simulink subsystem "Propagate_States"  (R2025b)
settings: Solver=VariableStepAuto  StartTime=0.0  StopTime=10.0  RelTol=1e-3
undefined symbols (not defined in the file): alt, g0, Ixx, Ixz, Iyy, Izz, Mass, p0, Phi0, Psi0, q0, r0, Theta0, u0, v0, w0
libraries: aerolibutil x1
settings Model: Creator=cdriggs  LastModifiedBy=cdriggs

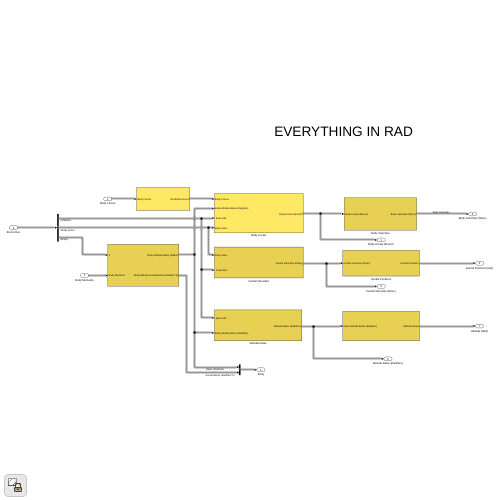
[thumbnail: Simulink's stored preview of the top-level diagram]
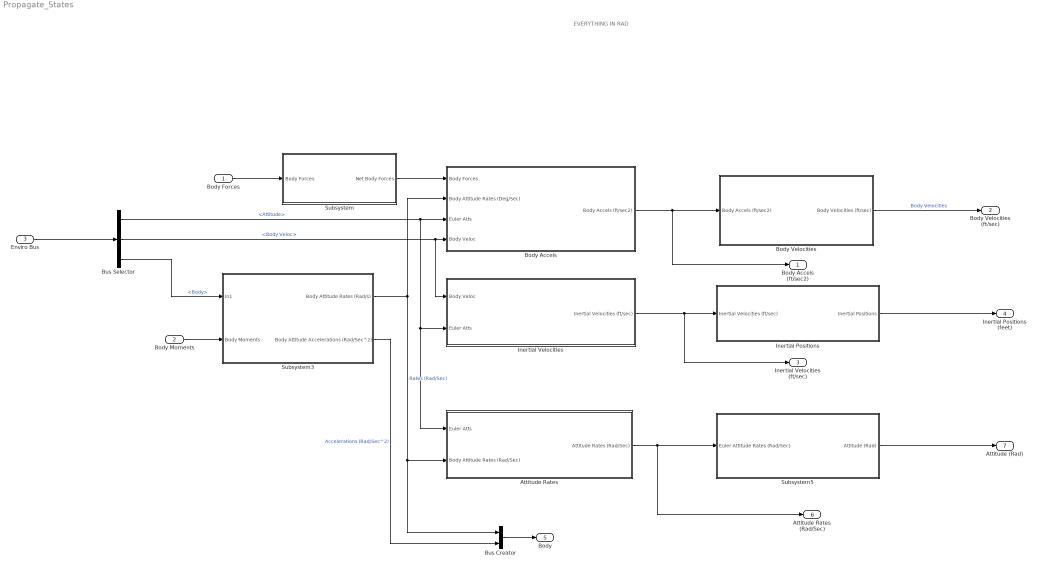
== system Propagate_States ==
  note: EVERYTHING IN RAD
  Body Forces : Inport
  Body Moments : Inport  Port=2
  Enviro Bus : Inport  Port=3
  Attitude Rates : Subsystem
  Body Accels : Subsystem
  Body Velocities : Subsystem
  Bus Creator : BusCreator  Inputs=2
  Bus Selector : BusSelector  OutputSignals=Rotat.Attitude,Trans.Body Veloc,Rotat.Body
  Inertial Positions : Subsystem
  Inertial Velocities : Subsystem
  Subsystem : Subsystem
  Subsystem3 : Subsystem
  Subsystem5 : Subsystem
  Body Accels (ft/sec2) : Outport
  Body Velocities (ft/sec) : Outport  Port=2
  Inertial Velocities (ft/sec) : Outport  Port=3
  Inertial Positions (feet) : Outport  Port=4
  " Body" : Outport  Port=5
  Attitude Rates (Rad/Sec) : Outport  Port=6
  Attitude (Rad) : Outport  Port=7
  wires:
  Bus Selector/3 -> Subsystem3/1(In1)  "<Body>"
  Bus Selector/2 -> Body Accels/4(Body Veloc), Inertial Velocities/1(Body Veloc)  "<Body Veloc>"
  Body Velocities/1(Body Velocities (ft/sec)) -> Body Velocities (ft/sec)/1  "Body Velocities"
  Subsystem3/1(Body Attitude Rates (Rad/s)) -> Body Accels/2(Body Attitude Rates (Deg/Sec)), Attitude Rates/2(Body Attitude Rates (Rad/Sec)), Bus Creator/1  "Rates (Rad/Sec)"
  Inertial Positions/1(Inertial Positions) -> Inertial Positions (feet)/1
  Inertial Velocities/1(Inertial Velocities (ft/sec)) -> Inertial Positions/1(Inertial Velocities (ft/sec)), Inertial Velocities (ft/sec)/1
  Body Accels/1(Body Accels (ft/sec2)) -> Body Velocities/1(Body Accels (ft/sec2)), Body Accels (ft/sec2)/1
  Body Moments/1 -> Subsystem3/2(Body Moments)
  Subsystem5/1(Attitude (Rad)) -> Attitude (Rad)/1
  Body Forces/1 -> Subsystem/1(Body Forces)
  Attitude Rates/1(Attitude Rates (Rad/Sec)) -> Attitude Rates (Rad/Sec)/1, Subsystem5/1(Euler Attitude Rates (Rad/Sec))
  Enviro Bus/1 -> Bus Selector/1
  Subsystem3/2(Body Attitude Accelerations (Rad/Sec^2)) -> Bus Creator/2  "Accelerations (Rad/Sec^2)"
  Subsystem/1(Net Body Forces) -> Body Accels/1(Body Forces)
  Bus Selector/1 -> Body Accels/3(" Euler Atts"), Inertial Velocities/2("  Euler Atts"), Attitude Rates/1(" Euler Atts ")  "<Attitude>"
  Bus Creator/1 -> " Body"/1

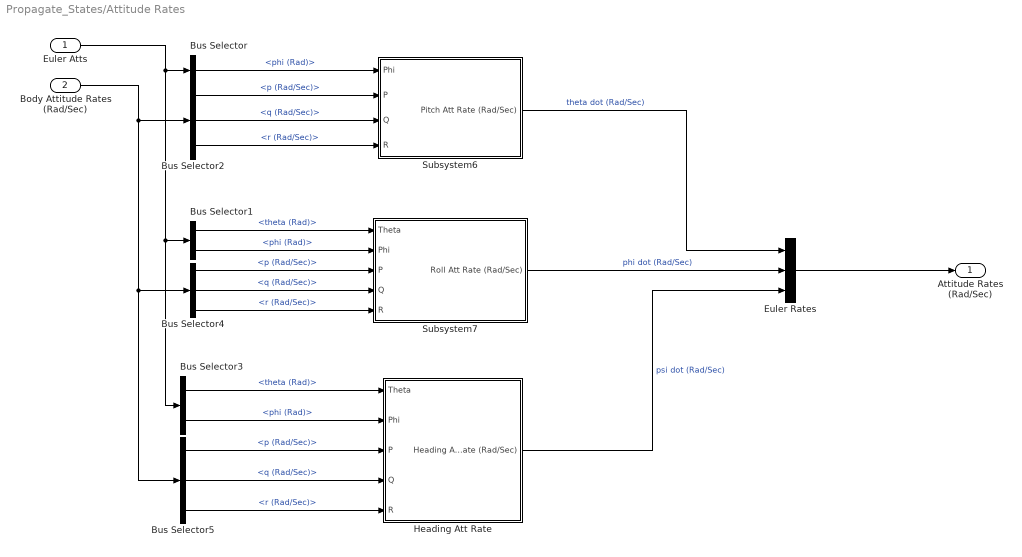
== system Propagate_States/Attitude Rates ==
  " Euler Atts " : Inport
  Body Attitude Rates (Rad/Sec) : Inport  Port=2
  Bus Selector : BusSelector  OutputSignals=phi (Rad)
  Bus Selector1 : BusSelector  OutputSignals=theta (Rad),phi (Rad)
  Bus Selector2 : BusSelector  OutputSignals=p (Rad/Sec),q (Rad/Sec),r (Rad/Sec)
  Bus Selector3 : BusSelector  OutputSignals=theta (Rad),phi (Rad)
  Bus Selector4 : BusSelector  OutputSignals=p (Rad/Sec),q (Rad/Sec),r (Rad/Sec)
  Bus Selector5 : BusSelector  OutputSignals=p (Rad/Sec),q (Rad/Sec),r (Rad/Sec)
  Euler Rates : BusCreator  Inputs=3
  Heading Att Rate : Subsystem
  Subsystem6 : Subsystem
  Subsystem7 : Subsystem
  Attitude Rates (Rad/Sec) : Outport
  wires:
  Bus Selector1/1 -> Subsystem7/1(Theta)  "<theta (Rad)>"
  Bus Selector1/2 -> Subsystem7/2(Phi)  "<phi (Rad)>"
  Bus Selector2/1 -> Subsystem6/2(P)  "<p (Rad/Sec)>"
  Bus Selector2/2 -> Subsystem6/3(Q)  "<q (Rad/Sec)>"
  Bus Selector2/3 -> Subsystem6/4(R)  "<r (Rad/Sec)>"
  Bus Selector4/1 -> Subsystem7/3(P)  "<p (Rad/Sec)>"
  Bus Selector4/2 -> Subsystem7/4(Q)  "<q (Rad/Sec)>"
  Bus Selector4/3 -> Subsystem7/5(R)  "<r (Rad/Sec)>"
  Euler Rates/1 -> Attitude Rates (Rad/Sec)/1
  Subsystem6/1(Pitch Att Rate (Rad/Sec)) -> Euler Rates/1  "theta dot (Rad/Sec)"
  Heading Att Rate/1(Heading Att Rate (Rad/Sec)) -> Euler Rates/3  "psi dot (Rad/Sec)"
  Subsystem7/1(Roll Att Rate (Rad/Sec)) -> Euler Rates/2  "phi dot (Rad/Sec)"
  Bus Selector/1 -> Subsystem6/1(Phi)  "<phi (Rad)>"
  Bus Selector3/1 -> Heading Att Rate/1(Theta)  "<theta (Rad)>"
  Bus Selector3/2 -> Heading Att Rate/2(Phi)  "<phi (Rad)>"
  " Euler Atts "/1 -> Bus Selector3/1, Bus Selector1/1, Bus Selector/1
  Bus Selector5/1 -> Heading Att Rate/3(P)  "<p (Rad/Sec)>"
  Body Attitude Rates (Rad/Sec)/1 -> Bus Selector5/1, Bus Selector4/1, Bus Selector2/1
  Bus Selector5/2 -> Heading Att Rate/4(Q)  "<q (Rad/Sec)>"
  Bus Selector5/3 -> Heading Att Rate/5(R)  "<r (Rad/Sec)>"

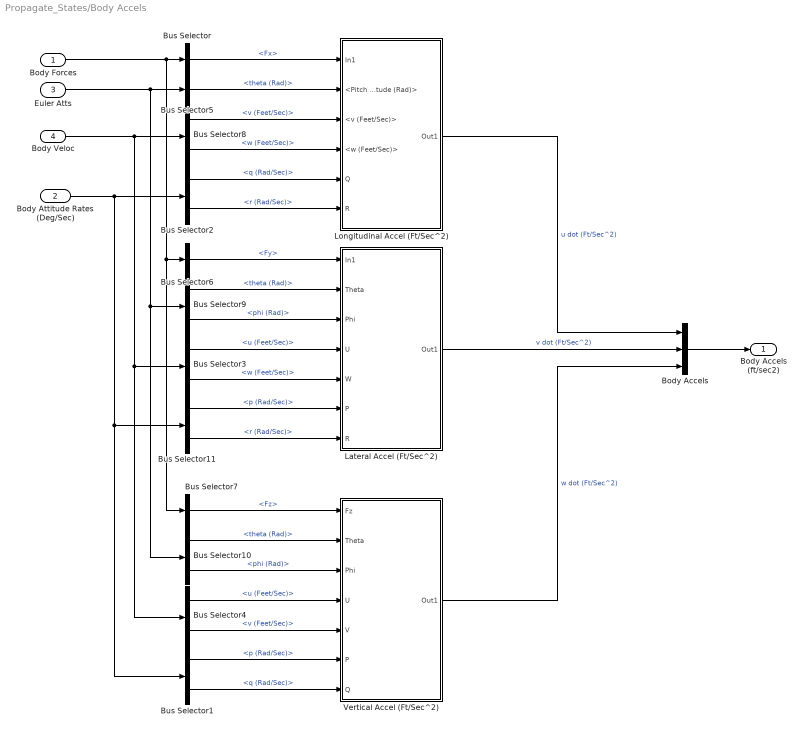
== system Propagate_States/Body Accels ==
  Body Forces : Inport
  Body Attitude Rates (Deg/Sec) : Inport  Port=2
  " Euler Atts" : Inport  Port=3
  Body Veloc : Inport  Port=4
  Body Accels : BusCreator  Inputs=3
  Bus Selector : BusSelector  OutputSignals=Fx
  Bus Selector1 : BusSelector  OutputSignals=p (Rad/Sec),q (Rad/Sec)
  Bus Selector10 : BusSelector  OutputSignals=theta (Rad),phi (Rad)
  Bus Selector11 : BusSelector  OutputSignals=p (Rad/Sec),r (Rad/Sec)
  Bus Selector2 : BusSelector  OutputSignals=q (Rad/Sec),r (Rad/Sec)
  Bus Selector3 : BusSelector  OutputSignals=u (Feet/Sec),w (Feet/Sec)
  Bus Selector4 : BusSelector  OutputSignals=u (Feet/Sec),v (Feet/Sec)
  Bus Selector5 : BusSelector  OutputSignals=theta (Rad)
  Bus Selector6 : BusSelector  OutputSignals=Fy
  Bus Selector7 : BusSelector  OutputSignals=Fz
  Bus Selector8 : BusSelector  OutputSignals=v (Feet/Sec),w (Feet/Sec)
  Bus Selector9 : BusSelector  OutputSignals=theta (Rad),phi (Rad)
  Lateral Accel (Ft/Sec^2) : Subsystem
  Longitudinal Accel (Ft/Sec^2) : Subsystem
  Vertical Accel (Ft/Sec^2) : Subsystem
  Body Accels (ft/sec2) : Outport
  wires:
  Bus Selector10/2 -> Vertical Accel (Ft/Sec^2)/3(Phi)  "<phi (Rad)>"
  Bus Selector10/1 -> Vertical Accel (Ft/Sec^2)/2(Theta)  "<theta (Rad)>"
  Bus Selector9/2 -> Lateral Accel (Ft/Sec^2)/3(Phi)  "<phi (Rad)>"
  Bus Selector9/1 -> Lateral Accel (Ft/Sec^2)/2(Theta)  "<theta (Rad)>"
  Bus Selector4/2 -> Vertical Accel (Ft/Sec^2)/5(V)  "<v (Feet/Sec)>"
  Bus Selector4/1 -> Vertical Accel (Ft/Sec^2)/4(U)  "<u (Feet/Sec)>"
  Bus Selector7/1 -> Vertical Accel (Ft/Sec^2)/1(Fz)  "<Fz>"
  Bus Selector6/1 -> Lateral Accel (Ft/Sec^2)/1(In1)  "<Fy>"
  Bus Selector3/1 -> Lateral Accel (Ft/Sec^2)/4(U)  "<u (Feet/Sec)>"
  Bus Selector3/2 -> Lateral Accel (Ft/Sec^2)/5(W)  "<w (Feet/Sec)>"
  Bus Selector8/2 -> Longitudinal Accel (Ft/Sec^2)/4(<w (Feet/Sec)>)  "<w (Feet/Sec)>"
  Bus Selector8/1 -> Longitudinal Accel (Ft/Sec^2)/3(<v (Feet/Sec)>)  "<v (Feet/Sec)>"
  Bus Selector5/1 -> Longitudinal Accel (Ft/Sec^2)/2(<Pitch Attitude (Rad)>)  "<theta (Rad)>"
  Bus Selector2/1 -> Longitudinal Accel (Ft/Sec^2)/5(Q)  "<q (Rad/Sec)>"
  Bus Selector2/2 -> Longitudinal Accel (Ft/Sec^2)/6(R)  "<r (Rad/Sec)>"
  Bus Selector1/2 -> Vertical Accel (Ft/Sec^2)/7(Q)  "<q (Rad/Sec)>"
  Bus Selector1/1 -> Vertical Accel (Ft/Sec^2)/6(P)  "<p (Rad/Sec)>"
  Body Attitude Rates (Deg/Sec)/1 -> Bus Selector11/1, Bus Selector1/1, Bus Selector2/1
  Bus Selector11/2 -> Lateral Accel (Ft/Sec^2)/7(R)  "<r (Rad/Sec)>"
  Bus Selector11/1 -> Lateral Accel (Ft/Sec^2)/6(P)  "<p (Rad/Sec)>"
  Bus Selector/1 -> Longitudinal Accel (Ft/Sec^2)/1(In1)  "<Fx>"
  Body Forces/1 -> Bus Selector/1, Bus Selector6/1, Bus Selector7/1
  " Euler Atts"/1 -> Bus Selector5/1, Bus Selector9/1, Bus Selector10/1
  Body Veloc/1 -> Bus Selector8/1, Bus Selector3/1, Bus Selector4/1
  Body Accels/1 -> Body Accels (ft/sec2)/1
  Longitudinal Accel (Ft/Sec^2)/1(Out1) -> Body Accels/1  "u dot (Ft/Sec^2)"
  Lateral Accel (Ft/Sec^2)/1(Out1) -> Body Accels/2  "v dot (Ft/Sec^2)"
  Vertical Accel (Ft/Sec^2)/1(Out1) -> Body Accels/3  "w dot (Ft/Sec^2)"

== system Propagate_States/Body Velocities ==
  Body Accels (ft/sec2) : Inport
  Body Velocities : BusCreator  Inputs=3
  Bus Selector : BusSelector  OutputSignals=u dot (Ft/Sec^2),v dot (Ft/Sec^2),w dot (Ft/Sec^2)
  Constant3 : Constant  Value=u0
  Constant4 : Constant  Value=v0
  Constant5 : Constant  Value=w0
  Integrator1 : Integrator  InitialConditionSource=external
  Integrator2 : Integrator  InitialConditionSource=external
  Integrator3 : Integrator  InitialConditionSource=external
  Pulse Generator : DiscretePulseGenerator  PulseType=Time based  Amplitude=50  Period=60  PulseWidth=5  PhaseDelay=2
  Sum : Sum  Inputs=|++
  Body Velocities (ft/sec) : Outport
  wires:
  Integrator3/1 -> Body Velocities/3  "w (Feet/Sec)"
  Pulse Generator/1 -> Sum/2
  Bus Selector/1 -> Integrator2/1  "<u dot (Ft/Sec^2)>"
  Body Accels (ft/sec2)/1 -> Bus Selector/1
  Bus Selector/2 -> Integrator1/1  "<v dot (Ft/Sec^2)>"
  Constant5/1 -> Integrator3/2
  Integrator2/1 -> Body Velocities/1  "u (Feet/Sec)"
  Constant3/1 -> Integrator2/2
  Bus Selector/3 -> Integrator3/1  "<w dot (Ft/Sec^2)>"
  Constant4/1 -> Integrator1/2
  Integrator1/1 -> Body Velocities/2  "v (Feet/Sec)"
  Body Velocities/1 -> Body Velocities (ft/sec)/1

== system Propagate_States/Inertial Positions ==
  Inertial Velocities (ft/sec) : Inport
  Bus Selector : BusSelector  OutputSignals=North-South Velocity (Feet/Sec),East-West Velocity (Feet/Sec),Inertial Vertical Speed (Feet/Sec)
  Constant : Constant  Value=0
  Constant1 : Constant  Value=0
  Constant2 : Constant  Value=-alt
  Inertial Positions ft : BusCreator  Inputs=3
  Integrator6 : Integrator  InitialConditionSource=external
  Integrator8 : Integrator  InitialConditionSource=external
  Integrator9 : Integrator  InitialConditionSource=external
  Inertial Positions : Outport
  wires:
  Constant1/1 -> Integrator8/2
  Constant/1 -> Integrator6/2
  Integrator8/1 -> Inertial Positions ft/2  "Longitude (Feet)"
  Inertial Positions ft/1 -> Inertial Positions/1
  Integrator6/1 -> Inertial Positions ft/1  "Latitude (Feet)"
  Inertial Velocities (ft/sec)/1 -> Bus Selector/1
  Bus Selector/1 -> Integrator6/1  "<North-South Velocity (Feet/Sec)>"
  Bus Selector/2 -> Integrator8/1  "<East-West Velocity (Feet/Sec)>"
  Bus Selector/3 -> Integrator9/1  "<Inertial Vertical Speed (Feet/Sec)>"
  Integrator9/1 -> Inertial Positions ft/3  "Inertial Altitude (Feet)"
  Constant2/1 -> Integrator9/2  "Inertial Altitude (Feet)"

== system Propagate_States/Inertial Velocities ==
  Body Veloc : Inport
  "  Euler Atts" : Inport  Port=2
  Bus Selector : BusSelector  OutputSignals=phi (Rad),theta (Rad),psi (Rad)
  Bus Selector1 : BusSelector  OutputSignals=phi (Rad),theta (Rad),psi (Rad)
  Bus Selector2 : BusSelector  OutputSignals=phi (Rad),theta (Rad)
  Bus Selector3 : BusSelector  OutputSignals=u (Feet/Sec),v (Feet/Sec),w (Feet/Sec)
  Bus Selector4 : BusSelector  OutputSignals=u (Feet/Sec),v (Feet/Sec),w (Feet/Sec)
  Bus Selector5 : BusSelector  OutputSignals=u (Feet/Sec),v (Feet/Sec),w (Feet/Sec)
  East-West Velocity (Feet/Sec) : Subsystem
  Inertial Velocities : BusCreator  Inputs=3
  Inertial Vertical Speed (Feet/Sec) : Subsystem
  North-South Velocity (Feet/Sec) : Subsystem
  Inertial Velocities (ft/sec) : Outport
  wires:
  "  Euler Atts"/1 -> Bus Selector2/1, Bus Selector1/1, Bus Selector/1
  Bus Selector/1 -> North-South Velocity (Feet/Sec)/1(Phi)  "<phi (Rad)>"
  Bus Selector/2 -> North-South Velocity (Feet/Sec)/2(Theta)  "<theta (Rad)>"
  Bus Selector/3 -> North-South Velocity (Feet/Sec)/3(Psi)  "<psi (Rad)>"
  Bus Selector1/1 -> East-West Velocity (Feet/Sec)/1(Phi)  "<phi (Rad)>"
  Bus Selector1/2 -> East-West Velocity (Feet/Sec)/2(Theta)  "<theta (Rad)>"
  Bus Selector1/3 -> East-West Velocity (Feet/Sec)/3(Psi)  "<psi (Rad)>"
  Bus Selector2/1 -> Inertial Vertical Speed (Feet/Sec)/1(Phi)  "<phi (Rad)>"
  Bus Selector2/2 -> Inertial Vertical Speed (Feet/Sec)/2(Theta)  "<theta (Rad)>"
  Body Veloc/1 -> Bus Selector5/1, Bus Selector4/1, Bus Selector3/1
  Bus Selector3/1 -> North-South Velocity (Feet/Sec)/4(U)  "<u (Feet/Sec)>"
  Bus Selector3/2 -> North-South Velocity (Feet/Sec)/5(V)  "<v (Feet/Sec)>"
  Bus Selector3/3 -> North-South Velocity (Feet/Sec)/6(W)  "<w (Feet/Sec)>"
  Bus Selector4/1 -> East-West Velocity (Feet/Sec)/4(U)  "<u (Feet/Sec)>"
  Bus Selector4/2 -> East-West Velocity (Feet/Sec)/5(V)  "<v (Feet/Sec)>"
  Bus Selector4/3 -> East-West Velocity (Feet/Sec)/6(W)  "<w (Feet/Sec)>"
  Bus Selector5/1 -> Inertial Vertical Speed (Feet/Sec)/3(U)  "<u (Feet/Sec)>"
  Bus Selector5/2 -> Inertial Vertical Speed (Feet/Sec)/4(V)  "<v (Feet/Sec)>"
  Bus Selector5/3 -> Inertial Vertical Speed (Feet/Sec)/5(W)  "<w (Feet/Sec)>"
  Inertial Velocities/1 -> Inertial Velocities (ft/sec)/1
  North-South Velocity (Feet/Sec)/1(North-South Velocity (Feet/Sec)) -> Inertial Velocities/1  "North-South Velocity (Feet/Sec)"
  East-West Velocity (Feet/Sec)/1(East-West Velocity (Feet/Sec)) -> Inertial Velocities/2  "East-West Velocity (Feet/Sec)"
  Inertial Vertical Speed (Feet/Sec)/1(Inertial Vertical Speed (Feet/Sec)) -> Inertial Velocities/3  "Inertial Vertical Speed (Feet/Sec)"

== system Propagate_States/Subsystem ==
  Body Forces : Inport
  Add1 : Sum
  Add2 : Sum
  Add3 : Sum
  Bus Creator : BusCreator  Inputs=3
  Bus Selector2 : BusSelector  OutputSignals=FAX (Lb),FTX (Lb),FAY (Lb),FTY (Lb),FAZ (Lb),FTZ (Lb)
  Net Body Forces : Outport
  wires:
  Add3/1 -> Bus Creator/3  "Fz"
  Bus Creator/1 -> Net Body Forces/1  "Net Body Forces"
  Bus Selector2/6 -> Add3/2  "<FTZ (Lb)>"
  Bus Selector2/5 -> Add3/1  "<FAZ (Lb)>"
  Bus Selector2/2 -> Add2/2  "<FTX (Lb)>"
  Bus Selector2/1 -> Add2/1  "<FAX (Lb)>"
  Add1/1 -> Bus Creator/2  "Fy"
  Add2/1 -> Bus Creator/1  "Fx"
  Bus Selector2/4 -> Add1/2  "<FTY (Lb)>"
  Body Forces/1 -> Bus Selector2/1
  Bus Selector2/3 -> Add1/1  "<FAY (Lb)>"

== system Propagate_States/Subsystem3 ==
  In1 : Inport
  Body Moments : Inport  Port=2
  Bus Selector9 : BusSelector  OutputSignals=Rates (Rad/Sec).p (Rad/Sec),Rates (Rad/Sec).q (Rad/Sec),Rates (Rad/Sec).r (Rad/Sec)
  Constant : Constant  Value=[Ixx 0 -Ixz; 0 Iyy 0; -Ixz 0 Izz]
  Invert 3x3 Matrix : aerolibutil/Invert  3x3 Matrix
  Make Vector 1 : Concatenate  NumInputs=3
  Make vector rows : Subsystem
  MatrixMultiply : Product  Multiplication=Matrix(*)
  Subsystem1 : Subsystem
  Subsystem4 : Subsystem
  Subsystem5 : Subsystem
  Body Attitude Rates (Rad/s) : Outport
  Body Attitude Accelerations (Rad/Sec^2) : Outport  Port=2
  wires:
  Body Moments/1 -> Subsystem5/1(Body Moments)
  Bus Selector9/3 -> Subsystem4/3(<Yaw Rate (Rad/Sec)>)  "<r (Rad/Sec)>"
  Bus Selector9/2 -> Subsystem4/2(<Pitch Rate (Rad/Sec)>)  "<q (Rad/Sec)>"
  Bus Selector9/1 -> Subsystem4/1(<Roll Rate (Rad/Sec)>)  "<p (Rad/Sec)>"
  Constant/1 -> Invert 3x3 Matrix/1
  In1/1 -> Bus Selector9/1
  Invert 3x3 Matrix/1 -> MatrixMultiply/1
  Make vector rows/1(Out1) -> Make Vector 1/1
  Make vector rows/2(Out2) -> Make Vector 1/2
  Make vector rows/3(Out3) -> Make Vector 1/3
  Make Vector 1/1 -> MatrixMultiply/2
  Subsystem4/3(QR) -> Make vector rows/3(QR)
  Subsystem4/4((P^2-R^2)) -> Make vector rows/4((P^2-R^2))
  Subsystem4/2(PR) -> Make vector rows/2(PR)
  Subsystem4/1(PQ) -> Make vector rows/1(PQ)
  Subsystem1/2(Body Attitude Accelerations (Rad/Sec^2)) -> Body Attitude Accelerations (Rad/Sec^2)/1
  Subsystem1/1(Body Attitude Rates (Rad/Sec)) -> Body Attitude Rates (Rad/s)/1
  MatrixMultiply/1 -> Subsystem1/1(In1)
  Subsystem5/1(Net Body Moments) -> Make vector rows/5(Net Body Moments)

== system Propagate_States/Subsystem5 ==
  Euler Attitude Rates (Rad/Sec) : Inport
  Bus Selector : BusSelector  OutputSignals=phi dot (Rad/Sec),theta dot (Rad/Sec),psi dot (Rad/Sec)
  Constant12 : Constant  Value=Psi0
  Constant14 : Constant  Value=Phi0
  Constant7 : Constant  Value=Theta0
  Euler Attitudes : BusCreator  Inputs=3
  Integrator4 : Integrator  InitialConditionSource=external
  Integrator5 : Integrator  InitialConditionSource=external
  Integrator7 : Integrator  InitialConditionSource=external
  Attitude (Rad) : Outport
  wires:
  Integrator5/1 -> Euler Attitudes/2  "theta (Rad)"
  Constant12/1 -> Integrator4/2
  Constant14/1 -> Integrator7/2
  Euler Attitude Rates (Rad/Sec)/1 -> Bus Selector/1
  Bus Selector/1 -> Integrator7/1  "<phi dot (Rad/Sec)>"
  Bus Selector/2 -> Integrator5/1  "<theta dot (Rad/Sec)>"
  Bus Selector/3 -> Integrator4/1  "<psi dot (Rad/Sec)>"
  Euler Attitudes/1 -> Attitude (Rad)/1
  Integrator4/1 -> Euler Attitudes/3  "psi (Rad)"
  Integrator7/1 -> Euler Attitudes/1  "phi (Rad)"
  Constant7/1 -> Integrator5/2

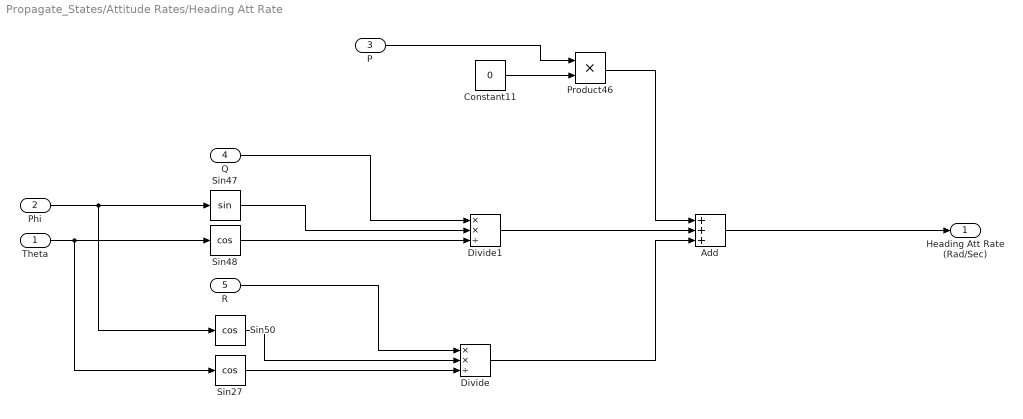
== system Propagate_States/Attitude Rates/Heading Att Rate ==
  Theta : Inport
  Phi : Inport  Port=2
  P : Inport  Port=3
  Q : Inport  Port=4
  R : Inport  Port=5
  Add : Sum  Inputs=+++
  Constant11 : Constant  Value=0
  Divide : Product  Inputs=**/
  Divide1 : Product  Inputs=**/
  Product46 : Product
  Sin27 : Trigonometry  Operator=cos
  Sin47 : Trigonometry
  Sin48 : Trigonometry  Operator=cos
  Sin50 : Trigonometry  Operator=cos
  Heading Att Rate (Rad/Sec) : Outport
  wires:
  Constant11/1 -> Product46/2
  Divide1/1 -> Add/2
  Divide/1 -> Add/3
  Sin50/1 -> Divide/2
  Sin48/1 -> Divide1/3
  Product46/1 -> Add/1
  Sin47/1 -> Divide1/2
  Sin27/1 -> Divide/3
  P/1 -> Product46/1
  Phi/1 -> Sin50/1, Sin47/1
  Theta/1 -> Sin27/1, Sin48/1
  R/1 -> Divide/1
  Add/1 -> Heading Att Rate (Rad/Sec)/1
  Q/1 -> Divide1/1

== system Propagate_States/Attitude Rates/Subsystem6 ==
  note: phi
  Phi : Inport
  P : Inport  Port=2
  Q : Inport  Port=3
  R : Inport  Port=4
  Add : Sum  Inputs=+++
  Constant9 : Constant  Value=0
  Gain : Gain  Gain=-1
  Product38 : Product
  Product39 : Product
  Product42 : Product
  Sin25 : Trigonometry  Operator=cos
  Sin26 : Trigonometry
  Pitch Att Rate (Rad/Sec) : Outport
  wires:
  Sin25/1 -> Product39/2
  Sin26/1 -> Gain/1
  Product42/1 -> Add/3
  Product38/1 -> Add/1
  Constant9/1 -> Product38/1
  Product39/1 -> Add/2
  P/1 -> Product38/2
  Q/1 -> Product39/1
  Phi/1 -> Sin26/1, Sin25/1
  R/1 -> Product42/1
  Add/1 -> Pitch Att Rate (Rad/Sec)/1  "Roll Att Rate (Rad/Sec)"
  Gain/1 -> Product42/2

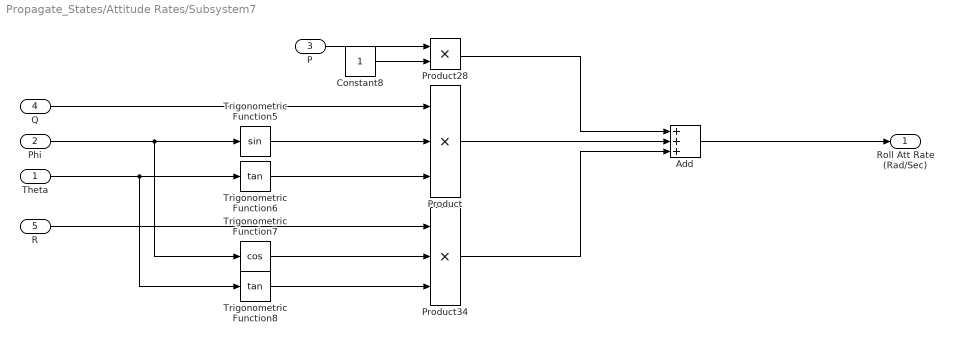
== system Propagate_States/Attitude Rates/Subsystem7 ==
  Theta : Inport
  Phi : Inport  Port=2
  P : Inport  Port=3
  Q : Inport  Port=4
  R : Inport  Port=5
  Add : Sum  Inputs=+++
  Constant8 : Constant
  Product : Product  Inputs=3
  Product28 : Product
  Product34 : Product  Inputs=3
  Trigonometric Function5 : Trigonometry
  Trigonometric Function6 : Trigonometry  Operator=tan
  Trigonometric Function7 : Trigonometry  Operator=cos
  Trigonometric Function8 : Trigonometry  Operator=tan
  Roll Att Rate (Rad/Sec) : Outport
  wires:
  Phi/1 -> Trigonometric Function7/1, Trigonometric Function5/1
  Theta/1 -> Trigonometric Function8/1, Trigonometric Function6/1
  P/1 -> Product28/1
  Product/1 -> Add/2
  Trigonometric Function8/1 -> Product34/3
  Trigonometric Function6/1 -> Product/3
  Constant8/1 -> Product28/2
  Product34/1 -> Add/3
  Trigonometric Function7/1 -> Product34/2
  R/1 -> Product34/1
  Trigonometric Function5/1 -> Product/2
  Product28/1 -> Add/1
  Add/1 -> Roll Att Rate (Rad/Sec)/1
  Q/1 -> Product/1

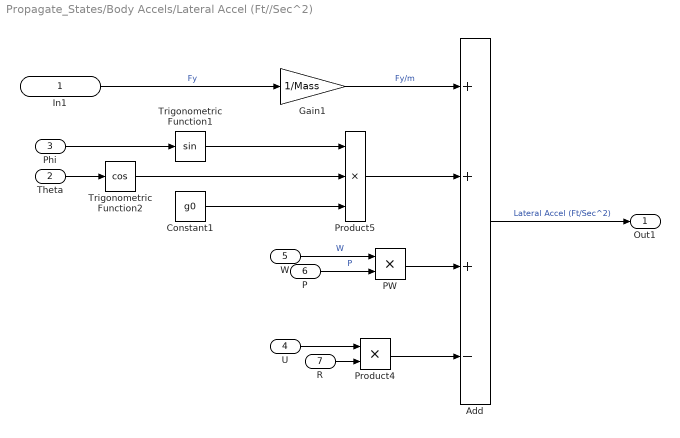
== system Propagate_States/Body Accels/Lateral Accel (Ft//Sec^2) ==
  In1 : Inport
  Theta : Inport  Port=2
  Phi : Inport  Port=3
  U : Inport  Port=4
  W : Inport  Port=5
  P : Inport  Port=6
  R : Inport  Port=7
  Add : Sum  Inputs=+++-
  Constant1 : Constant  Value=g0
  Gain1 : Gain  Gain=1/Mass
  PW : Product
  Product4 : Product
  Product5 : Product  Inputs=3
  Trigonometric Function1 : Trigonometry
  Trigonometric Function2 : Trigonometry  Operator=cos
  Out1 : Outport
  wires:
  Product5/1 -> Add/2
  Trigonometric Function1/1 -> Product5/1
  PW/1 -> Add/3
  Constant1/1 -> Product5/3
  In1/1 -> Gain1/1  "Fy"
  Trigonometric Function2/1 -> Product5/2
  Add/1 -> Out1/1  "Lateral Accel (Ft/Sec^2)"
  Product4/1 -> Add/4
  Phi/1 -> Trigonometric Function1/1
  Theta/1 -> Trigonometric Function2/1
  W/1 -> PW/1  "W"
  P/1 -> PW/2  "P"
  U/1 -> Product4/1
  R/1 -> Product4/2
  Gain1/1 -> Add/1  "Fy/m"

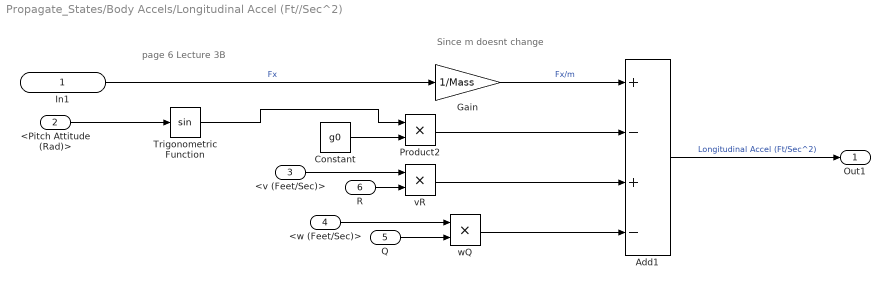
== system Propagate_States/Body Accels/Longitudinal Accel (Ft//Sec^2) ==
  note: page 6 Lecture 3B
  note: Since m doesnt change
  In1 : Inport
  <Pitch Attitude (Rad)> : Inport  Port=2
  <v (Feet/Sec)> : Inport  Port=3
  <w (Feet/Sec)> : Inport  Port=4
  Q : Inport  Port=5
  R : Inport  Port=6
  Add1 : Sum  Inputs=+-+-
  Constant : Constant  Value=g0
  Gain : Gain  Gain=1/Mass
  Product2 : Product
  Trigonometric Function : Trigonometry
  vR : Product
  wQ : Product
  Out1 : Outport
  wires:
  <Pitch Attitude (Rad)>/1 -> Trigonometric Function/1
  Trigonometric Function/1 -> Product2/1
  vR/1 -> Add1/3
  Gain/1 -> Add1/1  "Fx/m"
  Constant/1 -> Product2/2
  wQ/1 -> Add1/4
  In1/1 -> Gain/1  "Fx"
  Product2/1 -> Add1/2
  Add1/1 -> Out1/1  "Longitudinal Accel (Ft/Sec^2)"
  <v (Feet/Sec)>/1 -> vR/1
  R/1 -> vR/2
  <w (Feet/Sec)>/1 -> wQ/1
  Q/1 -> wQ/2

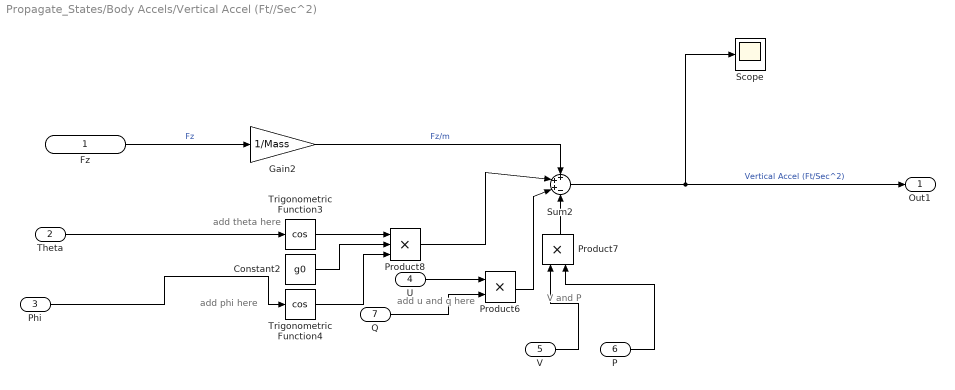
== system Propagate_States/Body Accels/Vertical Accel (Ft//Sec^2) ==
  note: add theta here
  note: V and P
  note: add u and q here
  note: add phi here
  Fz : Inport
  Theta : Inport  Port=2
  Phi : Inport  Port=3
  U : Inport  Port=4
  V : Inport  Port=5
  P : Inport  Port=6
  Q : Inport  Port=7
  Constant2 : Constant  Value=g0
  Gain2 : Gain  Gain=1/Mass
  Product6 : Product
  Product7 : Product
  Product8 : Product  Inputs=3
  Scope : Scope
      settings: ActiveDisplayYMinimum=-17.94081319561279  ActiveDisplayYMaximum=11.502802243959533  DataLoggingVariableName=ScopeData10
  Sum2 : Sum  Inputs=+++-
  Trigonometric Function3 : Trigonometry  Operator=cos
  Trigonometric Function4 : Trigonometry  Operator=cos
  Out1 : Outport
  wires:
  Fz/1 -> Gain2/1  "Fz"
  Constant2/1 -> Product8/2
  Product8/1 -> Sum2/2
  Product6/1 -> Sum2/3
  Trigonometric Function4/1 -> Product8/3
  Trigonometric Function3/1 -> Product8/1
  Gain2/1 -> Sum2/1  "Fz/m"
  Sum2/1 -> Out1/1, Scope/1  "Vertical Accel (Ft/Sec^2)"
  Product7/1 -> Sum2/4
  Theta/1 -> Trigonometric Function3/1
  Phi/1 -> Trigonometric Function4/1
  U/1 -> Product6/1
  Q/1 -> Product6/2
  V/1 -> Product7/1
  P/1 -> Product7/2

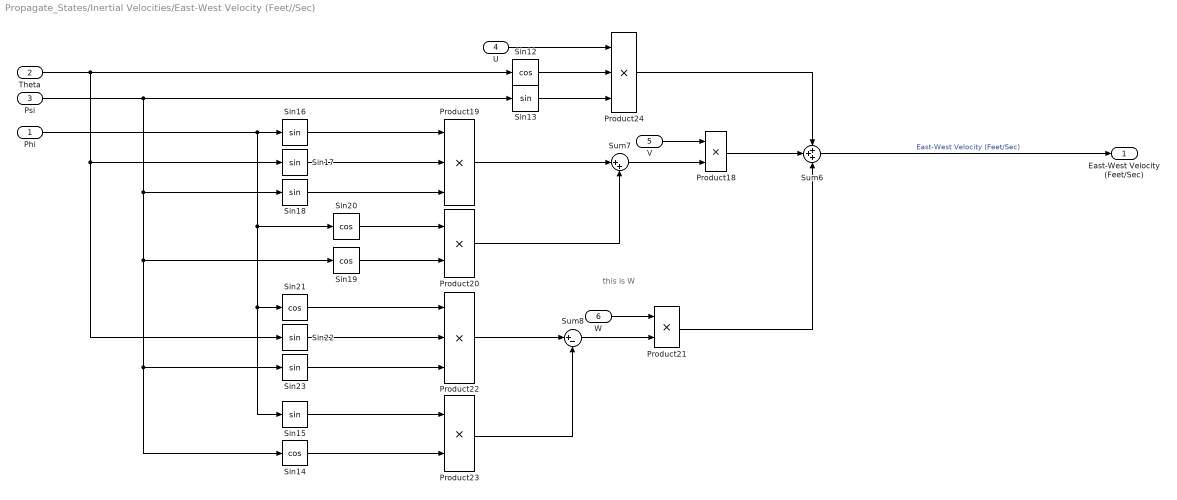
== system Propagate_States/Inertial Velocities/East-West Velocity (Feet//Sec) ==
  note: this is W
  Phi : Inport
  Theta : Inport  Port=2
  Psi : Inport  Port=3
  U : Inport  Port=4
  V : Inport  Port=5
  W : Inport  Port=6
  Product{18,20..21,23} (4 alike) : Product
  Product19 : Product  Inputs=3
  Product22 : Product  Inputs=3
  Product24 : Product  Inputs=3
  Sin{12,14,19..21} (5 alike) : Trigonometry  Operator=cos
  Sin{13,15..18,22..23} (7 alike) : Trigonometry
  Sum6 : Sum  Inputs=+++
  Sum7 : Sum  Inputs=|++
  Sum8 : Sum  Inputs=|+-
  East-West Velocity (Feet/Sec) : Outport
  wires:
  Sin14/1 -> Product23/2
  Sin17/1 -> Product19/2
  Sin15/1 -> Product23/1
  Product24/1 -> Sum6/1
  Product19/1 -> Sum7/1
  Sin22/1 -> Product22/2
  Product20/1 -> Sum7/2
  Product23/1 -> Sum8/2
  Sin16/1 -> Product19/1
  Sum7/1 -> Product18/2
  Sin12/1 -> Product24/2
  Product18/1 -> Sum6/2
  Sin23/1 -> Product22/3
  Sum8/1 -> Product21/2
  Product21/1 -> Sum6/3
  Sin21/1 -> Product22/1
  Product22/1 -> Sum8/1
  Sin13/1 -> Product24/3
  Sin18/1 -> Product19/3
  Sin19/1 -> Product20/2
  Sin20/1 -> Product20/1
  Sum6/1 -> East-West Velocity (Feet/Sec)/1  "East-West Velocity (Feet/Sec)"
  Phi/1 -> Sin21/1, Sin15/1, Sin20/1, Sin16/1
  Theta/1 -> Sin22/1, Sin17/1, Sin12/1
  Psi/1 -> Sin14/1, Sin23/1, Sin19/1, Sin18/1, Sin13/1
  U/1 -> Product24/1
  V/1 -> Product18/1
  W/1 -> Product21/1

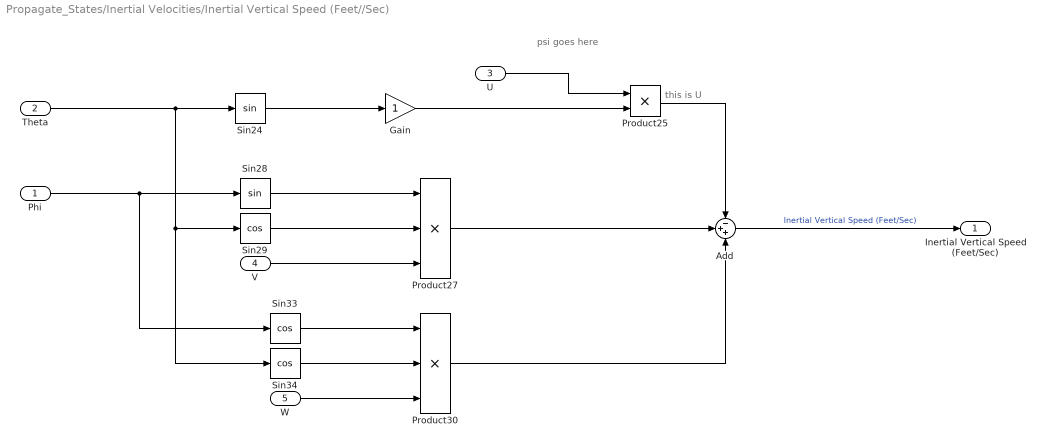
== system Propagate_States/Inertial Velocities/Inertial Vertical Speed (Feet//Sec) ==
  note: this is U
  note: psi goes here
  Phi : Inport
  Theta : Inport  Port=2
  U : Inport  Port=3
  V : Inport  Port=4
  W : Inport  Port=5
  Add : Sum  Inputs=-++
  Gain : Gain
  Product25 : Product
  Product27 : Product  Inputs=3
  Product30 : Product  Inputs=3
  Sin24 : Trigonometry
  Sin28 : Trigonometry
  Sin29 : Trigonometry  Operator=cos
  Sin33 : Trigonometry  Operator=cos
  Sin34 : Trigonometry  Operator=cos
  Inertial Vertical Speed (Feet/Sec) : Outport
  wires:
  Sin24/1 -> Gain/1
  Product30/1 -> Add/3
  Product25/1 -> Add/1
  Sin34/1 -> Product30/2
  Sin29/1 -> Product27/2
  Sin28/1 -> Product27/1
  Product27/1 -> Add/2
  Sin33/1 -> Product30/1
  Add/1 -> Inertial Vertical Speed (Feet/Sec)/1  "Inertial Vertical Speed (Feet/Sec)"
  Theta/1 -> Sin34/1, Sin29/1, Sin24/1
  Phi/1 -> Sin33/1, Sin28/1
  U/1 -> Product25/1
  W/1 -> Product30/3
  V/1 -> Product27/3
  Gain/1 -> Product25/2

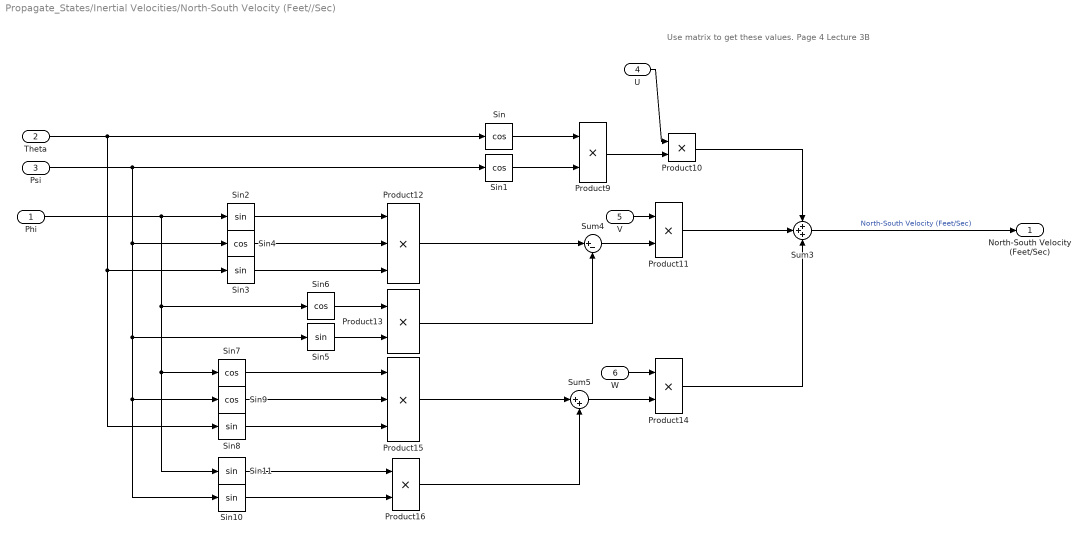
== system Propagate_States/Inertial Velocities/North-South Velocity (Feet//Sec) ==
  note: Use matrix to get these values. Page 4 Lecture 3B
  Phi : Inport
  Theta : Inport  Port=2
  Psi : Inport  Port=3
  U : Inport  Port=4
  V : Inport  Port=5
  W : Inport  Port=6
  Product{9..11,13..14,16} (6 alike) : Product
  Product12 : Product  Inputs=3
  Product15 : Product  Inputs=3
  Sin{,1,4,6..7,9} (6 alike) : Trigonometry  Operator=cos
  Sin{2..3,5,8,10..11} (6 alike) : Trigonometry
  Sum3 : Sum  Inputs=+++
  Sum4 : Sum  Inputs=|+-
  Sum5 : Sum  Inputs=|++
  North-South Velocity (Feet/Sec) : Outport
  wires:
  Sin6/1 -> Product13/1
  Sin7/1 -> Product15/1
  Sin10/1 -> Product16/2
  Product15/1 -> Sum5/1
  Product13/1 -> Sum4/2
  Product16/1 -> Sum5/2
  Sin/1 -> Product9/1
  Product10/1 -> Sum3/1
  Product14/1 -> Sum3/3
  Product9/1 -> Product10/2
  Product11/1 -> Sum3/2
  Product12/1 -> Sum4/1
  Sum4/1 -> Product11/2
  Sin5/1 -> Product13/2
  Sin11/1 -> Product16/1
  Sin2/1 -> Product12/1
  Sin1/1 -> Product9/2
  Sum5/1 -> Product14/2
  Sum3/1 -> North-South Velocity (Feet/Sec)/1  "North-South Velocity (Feet/Sec)"
  Phi/1 -> Sin2/1, Sin11/1, Sin7/1, Sin6/1
  Psi/1 -> Sin5/1, Sin10/1, Sin9/1, Sin4/1, Sin1/1
  Theta/1 -> Sin8/1, Sin3/1, Sin/1
  U/1 -> Product10/1
  V/1 -> Product11/1
  W/1 -> Product14/1
  Sin9/1 -> Product15/2
  Sin8/1 -> Product15/3
  Sin4/1 -> Product12/2
  Sin3/1 -> Product12/3

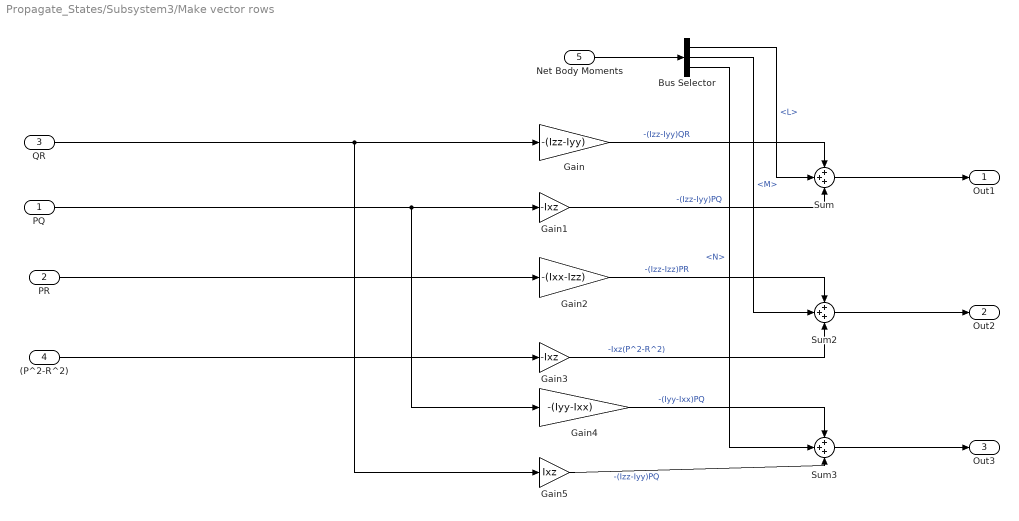
== system Propagate_States/Subsystem3/Make vector rows ==
  PQ : Inport
  PR : Inport  Port=2
  QR : Inport  Port=3
  (P^2-R^2) : Inport  Port=4
  Net Body Moments : Inport  Port=5
  Bus Selector : BusSelector  OutputSignals=L,M,N
  Gain : Gain  Gain=-(Izz-Iyy)
  Gain1 : Gain  Gain=-Ixz
  Gain2 : Gain  Gain=-(Ixx-Izz)
  Gain3 : Gain  Gain=-Ixz
  Gain4 : Gain  Gain=-(Iyy-Ixx)
  Gain5 : Gain  Gain=Ixz
  Sum : Sum  Inputs=+++
  Sum2 : Sum  Inputs=+++
  Sum3 : Sum  Inputs=+++
  Out1 : Outport
  Out2 : Outport  Port=2
  Out3 : Outport  Port=3
  wires:
  Net Body Moments/1 -> Bus Selector/1
  Gain/1 -> Sum/1  "-(Izz-Iyy)QR"
  Sum2/1 -> Out2/1
  Gain4/1 -> Sum3/1  "-(Iyy-Ixx)PQ"
  QR/1 -> Gain5/1, Gain/1
  Gain2/1 -> Sum2/1  "-(Izz-Izz)PR"
  Gain5/1 -> Sum3/3  "-(Izz-Iyy)PQ"
  Gain3/1 -> Sum2/3  "-Ixz(P^2-R^2)"
  Gain1/1 -> Sum/3  "-(Izz-Iyy)PQ"
  PR/1 -> Gain2/1
  PQ/1 -> Gain4/1, Gain1/1
  Sum3/1 -> Out3/1
  Bus Selector/3 -> Sum3/2  "<N>"
  (P^2-R^2)/1 -> Gain3/1
  Bus Selector/2 -> Sum2/2  "<M>"
  Sum/1 -> Out1/1
  Bus Selector/1 -> Sum/2  "<L>"

== system Propagate_States/Subsystem3/Subsystem1 ==
  In1 : Inport
  Body Rates : BusCreator  Inputs=3
  Bus Creator : BusCreator  Inputs=3
  Constant6 : Constant  Value=p0
  Constant8 : Constant  Value=q0
  Constant9 : Constant  Value=r0
  Demux : Demux  Outputs=3
  Demux1 : Demux  Outputs=3
  Integrator : Integrator  InitialConditionSource=external
  Integrator10 : Integrator  InitialConditionSource=external
  Integrator11 : Integrator  InitialConditionSource=external
  Body Attitude Rates (Rad/Sec) : Outport
  Body Attitude Accelerations (Rad/Sec^2) : Outport  Port=2
  wires:
  Body Rates/1 -> Body Attitude Rates (Rad/Sec)/1  "Body Attitude Accelerations (Rad/Sec^2)"
  Constant8/1 -> Integrator10/2
  Constant6/1 -> Integrator/2
  Integrator/1 -> Body Rates/1  "p (Rad/Sec)"
  Integrator10/1 -> Body Rates/2  "q (Rad/Sec)"
  Integrator11/1 -> Body Rates/3  "r (Rad/Sec)"
  Constant9/1 -> Integrator11/2
  Bus Creator/1 -> Body Attitude Accelerations (Rad/Sec^2)/1  "Body Attitude Accelerations (Rad/Sec^2)"
  Demux1/2 -> Integrator10/1, Bus Creator/2  "q dot  (Rad/Sec^2)"
  Demux1/1 -> Integrator/1, Bus Creator/1  "p dot (Rad/Sec^2)"
  Demux1/3 -> Integrator11/1, Bus Creator/3  "r dot (Rad/Sec^2)"
  In1/1 -> Demux1/1

== system Propagate_States/Subsystem3/Subsystem4 ==
  <Roll Rate (Rad/Sec)> : Inport
  <Pitch Rate (Rad/Sec)> : Inport  Port=2
  <Yaw Rate (Rad/Sec)> : Inport  Port=3
  Product : Product
  Product1 : Product
  Product2 : Product
  Square : Math  Operator=square
  Square1 : Math  Operator=square
  Sum1 : Sum  Inputs=+|-
  PQ : Outport
  PR : Outport  Port=2
  QR : Outport  Port=3
  (P^2-R^2) : Outport  Port=4
  wires:
  <Pitch Rate (Rad/Sec)>/1 -> Product/2, Product1/1  "Q"
  <Roll Rate (Rad/Sec)>/1 -> Product/1, Product2/1, Square/1  "P"
  Product2/1 -> PR/1  "PR"
  <Yaw Rate (Rad/Sec)>/1 -> Product1/2, Square1/1, Product2/2  "R"
  Square1/1 -> Sum1/2  "R^2"
  Square/1 -> Sum1/1  "P^2"
  Sum1/1 -> (P^2-R^2)/1  "(P^2-R^2)"
  Product/1 -> PQ/1  "PQ"
  Product1/1 -> QR/1  "QR"

== system Propagate_States/Subsystem3/Subsystem5 ==
  Body Moments : Inport
  Add3 : Sum
  Add4 : Sum
  Add5 : Sum
  Bus Creator : BusCreator  Inputs=3
  Bus Selector3 : BusSelector  OutputSignals=MAY (Lb-Ft),MTY (Lb-Ft)
  Bus Selector5 : BusSelector  OutputSignals=MAZ (Lb-Ft),MTZ (Lb-Ft)
  Bus Selector8 : BusSelector  OutputSignals=MAX (Lb-Ft),MTX (Lb-Ft)
  Net Body Moments : Outport
  wires:
  Bus Creator/1 -> Net Body Moments/1  "Net Body Moments"
  Body Moments/1 -> Bus Selector8/1, Bus Selector5/1, Bus Selector3/1
  Bus Selector8/2 -> Add3/2  "<MTX (Lb-Ft)>"
  Bus Selector5/2 -> Add5/2  "<MTZ (Lb-Ft)>"
  Bus Selector3/2 -> Add4/2  "<MTY (Lb-Ft)>"
  Bus Selector8/1 -> Add3/1  "<MAX (Lb-Ft)>"
  Bus Selector5/1 -> Add5/1  "<MAZ (Lb-Ft)>"
  Bus Selector3/1 -> Add4/1  "<MAY (Lb-Ft)>"
  Add4/1 -> Bus Creator/2  "M"
  Add3/1 -> Bus Creator/1  "L"
  Add5/1 -> Bus Creator/3  "N"
